simulink model "PIDstatespace"  (R2023b)
settings: Solver=FixedStepAuto  StartTime=0  StopTime=10  FixedStep=0.01  RelTol=1e-3
undefined symbols (not defined in the file): A, B, C, D, Kd_alpha, Kd_theta, Ki_alpha, Ki_theta, Kp_alpha, Kp_theta
settings Model: Creator=lxy18  LastModifiedBy=lxy18

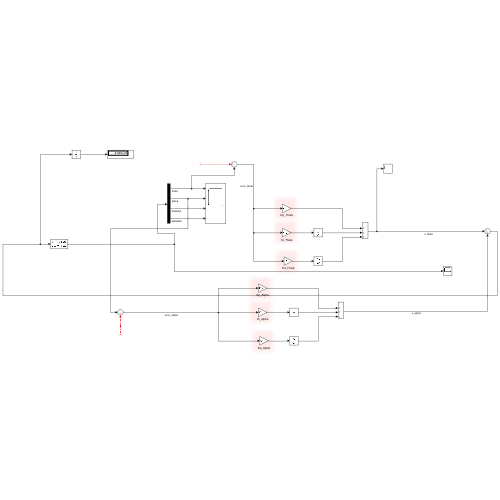
[thumbnail: Simulink's stored preview of the top-level diagram]
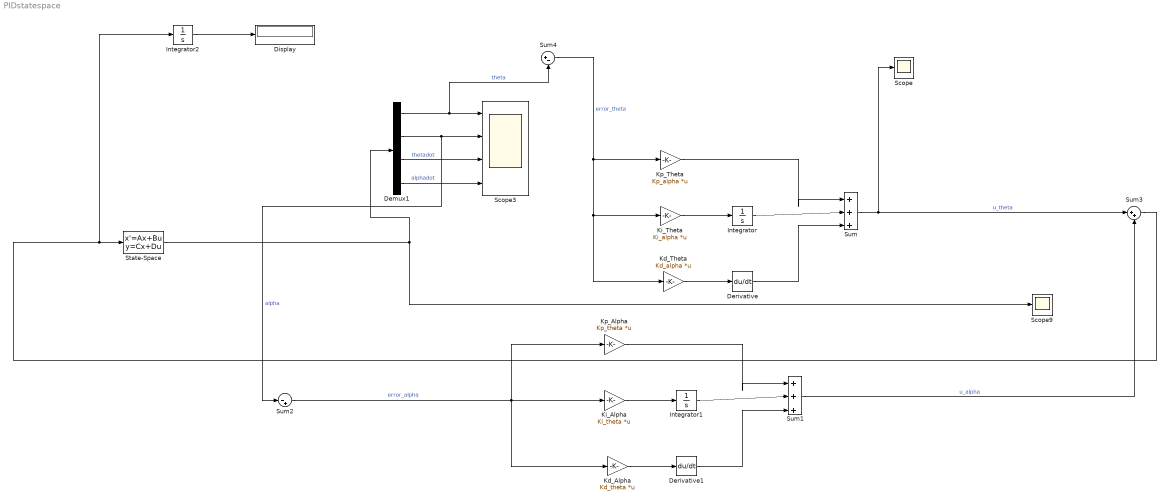
== system PIDstatespace ==
  Demux1 : Demux
  Derivative : Derivative
  Derivative1 : Derivative
  Display : Display
  Integrator : Integrator
  Integrator1 : Integrator
  Integrator2 : Integrator
  Kd_Alpha : Gain  Gain=Kd_theta  Multiplication=Matrix(K*u)
  Kd_Theta : Gain  Gain=Kd_alpha  Multiplication=Matrix(K*u)
  Ki_Alpha : Gain  Gain=Ki_theta  Multiplication=Matrix(K*u)
  Ki_Theta : Gain  Gain=Ki_alpha  Multiplication=Matrix(K*u)
  Kp_Alpha : Gain  Gain=Kp_theta  Multiplication=Matrix(K*u)
  Kp_Theta : Gain  Gain=Kp_alpha  Multiplication=Matrix(K*u)
  Scope : Scope
  Scope3 : Scope  NumInputPorts=4
  Scope9 : Scope
  State-Space : StateSpace  A=A  B=B  C=C  D=D  InitialCondition=[1 * pi / 180;1 * pi / 180;0;0]
  Sum : Sum  Inputs=|+++
  Sum1 : Sum  Inputs=|+++
  Sum2 : Sum  Inputs=|-+
  Sum3 : Sum  Inputs=|++
  Sum4 : Sum  Inputs=|+-
  wires:
  Kp_Alpha/1 -> Sum1/1
  Kd_Theta/1 -> Derivative/1
  Integrator/1 -> Sum/2
  Kp_Theta/1 -> Sum/1
  State-Space/1 -> Scope9/1, Demux1/1
  Integrator1/1 -> Sum1/2
  Derivative1/1 -> Sum1/3
  Ki_Alpha/1 -> Integrator1/1
  Derivative/1 -> Sum/3
  Ki_Theta/1 -> Integrator/1
  Kd_Alpha/1 -> Derivative1/1
  ? -> Sum4/1
  Sum4/1 -> Kp_Theta/1, Kd_Theta/1, Ki_Theta/1  "error_theta"
  Demux1/1 -> Sum4/2, Scope3/1  "theta"
  Demux1/2 -> Sum2/1, Scope3/2  "alpha"
  Demux1/3 -> Scope3/3  "thetadot"
  Demux1/4 -> Scope3/4  "alphadot"
  Sum2/1 -> Kd_Alpha/1, Kp_Alpha/1, Ki_Alpha/1  "error_alpha"
  ? -> Sum2/2
  Sum/1 -> Sum3/1, Scope/1  "u_theta"
  Sum1/1 -> Sum3/2  "u_alpha"
  Sum3/1 -> Integrator2/1, State-Space/1
  Integrator2/1 -> Display/1
